simulink model "PIDSO"  (R2014a)
settings: Solver=ode3  StartTime=0.0  StopTime=15  FixedStep=T  RelTol=1e-3
undefined symbols (not defined in the file or in its folder): Kp, T
libraries: simulink x1
settings Model: Creator=tri  LastModifiedBy=tri

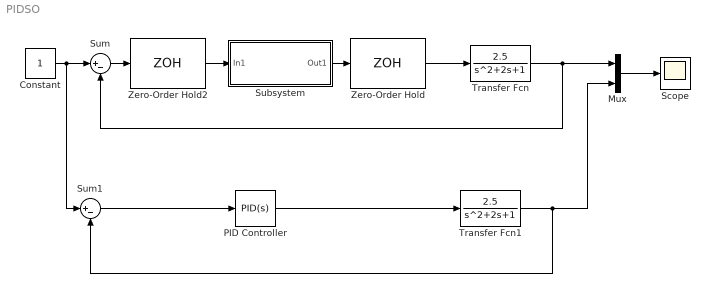
== system PIDSO ==
  Constant : Constant
  Mux : Mux  Inputs=2
  PID Controller : simulink/Continuous/PID Controller  Controller=PID  TimeDomain=Continuous-time  SampleTime=1  IntegratorMethod=Forward Euler  FilterMethod=Forward Euler  Form=Parallel  P=0.2  I=0.2  D=0  N=100  InitialConditionSource=internal  InitialConditionForIntegrator=0  InitialConditionForFilter=0  ExternalReset=none  LimitOutput=off  UpperSaturationLimit=inf  LowerSaturationLimit=-inf  LinearizeAsGain=on  AntiWindupMode=none  Kb=1  TrackingMode=off  Kt=1  PParamMin=[]  PParamMax=[]  IParamMin=[]  IParamMax=[]  DParamMin=[]  DParamMax=[]  NParamMin=[]  NParamMax=[]  KbParamMin=[]  KbParamMax=[]  KtParamMin=[]  KtParamMax=[]  POutMin=[]  POutMax=[]  IOutMin=[]  IOutMax=[]  DOutMin=[]  DOutMax=[]  NOutMin=[]  NOutMax=[]  KbOutMin=[]  KbOutMax=[]  KtOutMin=[]  KtOutMax=[]  IntegratorOutMin=[]  IntegratorOutMax=[]  FilterOutMin=[]  FilterOutMax=[]  SumOutMin=[]  SumOutMax=[]  SumI1OutMin=[]  SumI1OutMax=[]  SumI2OutMin=[]  SumI2OutMax=[]  SumI3OutMin=[]  SumI3OutMax=[]  SumDOutMin=[]  SumDOutMax=[]  SaturationOutMin=[]  SaturationOutMax=[]  IntegratorContinuousStateAttributes=''  IntegratorStateMustResolveToSignalObject=off  IntegratorRTWStateStorageClass=Auto  FilterContinuousStateAttributes=''  FilterStateMustResolveToSignalObject=off  FilterRTWStateStorageClass=Auto
  Scope : Scope
      settings: YMin=0  YMax=2
  Subsystem : Subsystem
  Sum : Sum  Inputs=|+-
  Sum1 : Sum  Inputs=|+-
  Transfer Fcn : TransferFcn  Numerator=[2.5]
  Transfer Fcn1 : TransferFcn  Numerator=[2.5]
  Zero-Order Hold : ZeroOrderHold  SampleTime=T
  Zero-Order Hold2 : ZeroOrderHold  SampleTime=T
  wires:
  Constant/1 -> Sum1/1, Sum/1
  Subsystem/1(Out1) -> Zero-Order Hold/1
  Zero-Order Hold/1 -> Transfer Fcn/1
  Zero-Order Hold2/1 -> Subsystem/1(In1)
  Sum/1 -> Zero-Order Hold2/1
  PID Controller/1 -> Transfer Fcn1/1
  Transfer Fcn1/1 -> Mux/2, Sum1/2
  Sum1/1 -> PID Controller/1
  Mux/1 -> Scope/1
  Transfer Fcn/1 -> Mux/1, Sum/2

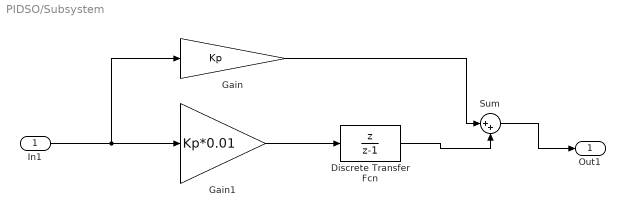
== system PIDSO/Subsystem ==
  In1 : Inport
  Discrete Transfer Fcn : DiscreteTransferFcn  Numerator=[1 0]  Denominator=[1 -1]  SampleTime=T
  Gain : Gain  Gain=Kp
  Gain1 : Gain  Gain=Kp*0.01
  Sum : Sum  Inputs=|++
  Out1 : Outport
  wires:
  Gain1/1 -> Discrete Transfer Fcn/1
  In1/1 -> Gain/1, Gain1/1
  Discrete Transfer Fcn/1 -> Sum/2
  Gain/1 -> Sum/1
  Sum/1 -> Out1/1
